simulink model "matmul"  (R2017a)
settings: Solver=VariableStepAuto  StartTime=0.0  StopTime=10.0  RelTol=1e-3
settings Model: Creator=HP  LastModifiedBy=HP

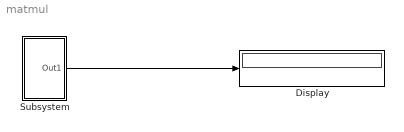
== system matmul ==
  Display : Display
  Subsystem : Subsystem
  wires:
  Subsystem/1(Out1) -> Display/1

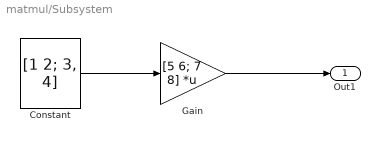
== system matmul/Subsystem ==
  Constant : Constant  Value=[1 2; 3, 4]
  Gain : Gain  Gain=[5 6; 7 8]  Multiplication=Matrix(K*u)
  Out1 : Outport
  wires:
  Constant/1 -> Gain/1
  Gain/1 -> Out1/1
